simulink model "EA_Model"  (R2023a)
settings: Solver=VariableStepAuto  StartTime=0.0  StopTime=inf  RelTol=1e-3
StartFcn:
  | 1
StopFcn:
  | 1
model workspace: external: MATLAB File H:\My Drive\MECH5108EnviSat\Original Design\EA_Model_DataFile.m (data not in the file)
values from neighbouring files (symbols this model uses):
  N = 10    [EA_Main.m]
  s = 3*((timeinterval*(i-1))/tf)^2-2*((timeinterval*(i-1))/tf)^3    [cartesian_traj_gen.m]
  timeinterval = time/(size(theta_matrix,1)-1)    [EA_Main.m]    (also in cartesian_traj_gen.m = tf/(N-1))
undefined symbols (not defined in the file or in its folder): smiData, X, Y, Z
libraries: sm_lib x44, nesl_utility x14
(part 2 of 2)

== matlab function EA_Model/MATLAB Function ==
  data: t input; tau_control output; dt input; tgoal input; dtgoal input; ddtgoal input; Kp input; Kd input
function tau_control = CTC(t,dt,tgoal, dtgoal, ddtgoal, Kp, Kd)
% Source: https://github.com/NxRLab/ModernRobotics/blob/master/packages/MATLAB/mr/ComputedTorque.m
g = [0;0;-9.8];

%Link Lengths
L0 = 0.7;
L1 = 0.3; 
L2 = 0.6;
L3 = 0.61;
L4 = 0.2;
L5 = 0.325;
L6 = 0.1;
EE = 0.2;

%Link Radii
rb = ((0.3+0.25)/2)/2;
rL1 = 0.25/2;
rL2 = 0.25/2;
rL3 = ((0.25+0.2)/2)/2;
rL4 = 0.2/2;
rL5 = 0.09/2;
rL6 = 0.16/2;


%Link Masses (kg)
m0 = 58.82122;
m1 = 12.14307;
m2 = 27.51008;
m3 = 22.95120;
m4 = 5.34717;
m5 = 3.18720;
m6 = 0.27655;

%Positions of the center of mass for each link
%Position of CoM for Link 1 with reference to World Frame (No rotation)
M0L1 = [1  0  0  0;
         0  1  0  0;
         0  0  1  L0+(L1/2);
         0  0  0  1];
%Position of CoM for Link 2 with reference to Link 1 (+ve y rotation by 90 degrees)
ML1L2 = [0  0  1  0;
         0  1  0  -L2/2;
         -1  0  0  L1/2;
         0  0  0  1];
%Position of CoM for Link 3 with reference to Link 2 (No rotation)
ML2L3 = [1  0  0  L3/2;
         0  1  0  -L2/2;
         0  0  1  0;
         0  0  0  1];
%Position of CoM for Link 4 with reference to Link 3 (+ve y rotation by 90 degrees)
ML3L4 = [0  0  1  (L3/2)+(L4/2);
         0  1  0  0;
        -1  0  0  0;
         0  0  0  1];
%Position of CoM for Link 5 with reference to Link 4 (-ve y rotation by 90 degrees)
ML4L5 = [0  0  -1  0;
         0  1  0  L5/2;
         1  0  0  L4/2;
         0  0  0  1];
%Position of CoM for Gripper Base with Reference to Link 5 (+ve x rotation by 90 degrees)
ML5L6 = [1  0  0  0;
         0  0  -1  (L5/2)+(L6/2);
         0  1  0  0;
         0  0  0  1];
%Position of End Effector with respect to Gripper Base (No Rotation)
ML6EE = [1  0  0  0;
        0  1  0  0;
        0  0  1  (L6/2)+ EE;
        0  0  0  1];

Ml = cat(3, M0L1, ML1L2, ML2L3, ML3L4, ML4L5, ML5L6, ML6EE);

%Defining the Inertia Matrices for Each Link
In1 = [m1*(3*rL1^2+L1^2)/12,m1*(3*rL1^2+L1^2)/12, (m1*rL1^2)/2];
In1m1 = [In1,m1,m1,m1];
In2 = [m2*(3*rL2^2+L2^2)/12,m2*(3*rL2^2+L2^2)/12, (m2*rL2^2)/2];
In2m2 = [In2,m2,m2,m2];
In3 = [m3*(3*rL3^2+L3^2)/12,m3*(3*rL3^2+L3^2)/12, (m3*rL3^2)/2];
In3m3 = [In3,m3,m3,m3];
In4 = [m4*(3*rL4^2+L4^2)/12,m4*(3*rL4^2+L4^2)/12, (m4*rL4^2)/2];
In4m4 = [In4,m4,m4,m4];
In5 = [m5*(3*rL5^2+L5^2)/12,m5*(3*rL5^2+L5^2)/12, (m5*rL5^2)/2];
In5m5 = [In5,m5,m5,m5];
In6 = [m6*(3*rL6^2+L6^2)/12,m6*(3*rL6^2+L6^2)/12, (m6*rL6^2)/2];
In6m6 = [In6,m6,m6,m6];

%Spatial Inertia Matrix for Each Link Relative to Corresponding Frames
G1 = diag(In1m1);
G2 = diag(In2m2);
G3 = diag(In3m3);
G4 = diag(In4m4);
G5 = diag(In5m5);
G6 = diag(In6m6);

Gl = cat(3, G1,G2,G3,G4,G5,G6);

%Screw Axes
% Determining the position and screw axis with respect to the end-effector
% for joint 1
a1 = [0; -L4-L3+L1+L0; -L5+L2]; %joint position
Bw1 = [0; -1; 0]; % angular component (-y)
Bv1 = cross(-Bw1,a1); %linear component
B1 = [Bw1; Bv1]; %Screw Axis

% Determining the position and screw axis with respect to the end-effector
% for joint 2
a2 = [0; -L4-L3; -L5+L2]; %joint position
Bw2 = [-1; 0; 0]; % angular component (-x)
Bv2 = cross(-Bw2,a2); %linear component
B2 = [Bw2; Bv2]; %Screw Axis

% Determining the position and screw axis with respect to the end-effector
% for joint 3
a3 = [0; -L4-L3; -L5]; %joint position
Bw3 = [-1; 0; 0];% angular component (-x)
Bv3 = cross(-Bw3,a3); %linear component
B3 = [Bw3; Bv3];%Screw Axis

% Determining the position and screw axis with respect to the end-effector
% for joint 4
a4 = [0; -L4; -L5];%joint position
Bw4 = [0; -1; 0]; % angular component (-y)
Bv4 = cross(-Bw4,a4);%linear component
B4 = [Bw4; Bv4]; %Screw Axis

% Determining the position and screw axis with respect to the end-effector
% for joint 5
a5 = [0; 0; -L5];%joint position
Bw5 = [-1; 0; 0]; % angular component (-x)
Bv5 = cross(-Bw5,a5);%linear component
B5 = [Bw5; Bv5];%Screw Axis

% Determining the position and screw axis with respect to the end-effector
% for joint 6
a6 = [0; 0; 0];%joint position
Bw6 = [0; 0; 1]; % angular component (+z)
Bv6 = cross(-Bw6,a6);%linear component
B6 = [Bw6; Bv6];%Screw Axis

%List of screw axes
Bl = [B1 B2 B3 B4 B5 B6];

err = tgoal - t;
if size(t,1) == 6
    % tau_control = Mmat(t, Ml, Gl, Bl)*(Kp * err + Kd * (dtgoal - dt)) + inv_dyn(t,dt,ddtgoal,g);
    tau_control = Mmat(t, Ml, Gl, Bl)*(Kp * err + Kd * (dtgoal - dt))+ inv_dyn(t,dt,ddtgoal,g);
    % tau_control(1)=0;
    % tau_control(3)=0;
    % tau_control(4)=0;
    % tau_control(5)=0;
    % tau_control(6)=0;
else 
    tau_control = [0;0;0;0;0;0];
end

end

function M = Mmat(t, Ml, Gl, Bl)
g = [0;0;0];
n = size(t,1);
M = zeros(n);
for i = 1:n
    ddt = zeros(n,1);
    ddt(i) = 1;
    M(:,i) = inv_dyn(t, zeros(n,1), ddt,g);
end
end
